simulink model "ADRC_ESO_feedback_comparison"  (R2020b)
settings: Solver=VariableStepAuto  StartTime=0.0  StopTime=10.0  RelTol=1e-3
values from neighbouring files (symbols this model uses):
  b = V*Km/(g*Tc^2*57.3)    [param_ADRC_ang_acc_change.m]
  b0 = -30    [param_ADRC_ang_acc_change.m]
  g = 9.81    [param_ADRC_ang_acc_change.m]
  g1 = 1/Tc^2    [param_ADRC_ang_acc_change.m]
  g2 = 2*Ac/Tc    [param_ADRC_ang_acc_change.m]
  kd = 2*wc*V/(g*57.3)    (= 21.3480207716)    [param_ADRC_ang_acc_change.m]
  kp = wc^2    (= 400)    [param_ADRC_ang_acc_change.m]
  V = 300    [param_ADRC_ang_acc_change.m]
  wo = 80    [param_ADRC_ang_acc_change.m]
settings Model: Creator=11814  LastModifiedBy=11814

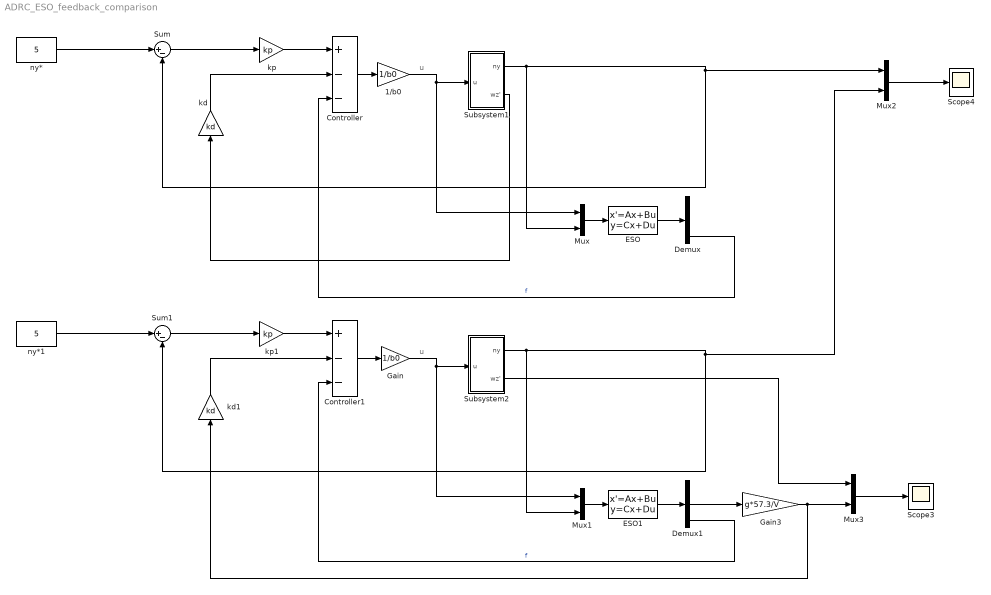
== system ADRC_ESO_feedback_comparison ==
  note: u
  note: u
  1/b0 : Gain  Gain=1/b0
  Controller : Sum  Inputs=+--
  Controller1 : Sum  Inputs=+--
  Demux : Demux  Outputs=3
  Demux1 : Demux  Outputs=3
  ESO : StateSpace  A=[-3*wo 1 0; -3*wo^2 0 1; -wo^3 0 0]  B=[0 3*wo; b0 3*wo^2; 0 wo^3]  C=eye(3)  D=[0 0; 0 0; 0 0]  InitialCondition=0
  ESO1 : StateSpace  A=[-3*wo 1 0; -3*wo^2 0 1; -wo^3 0 0]  B=[0 3*wo; b0 3*wo^2; 0 wo^3]  C=eye(3)  D=[0 0; 0 0; 0 0]  InitialCondition=0
  Gain : Gain  Gain=1/b0
  Gain3 : Gain  Gain=g*57.3/V
  Mux{,1..3} (4 alike) : Mux  Inputs=2
  Scope3 : Scope
  Scope4 : Scope
  Subsystem1 : Subsystem
  Subsystem2 : Subsystem
  Sum : Sum  Inputs=|+-
  Sum1 : Sum  Inputs=|+-
  kd : Gain  Gain=kd
  kd1 : Gain  Gain=kd
  kp : Gain  Gain=kp
  kp1 : Gain  Gain=kp
  ny* : Constant  Value=5
  ny*1 : Constant  Value=5
  wires:
  Controller/1 -> 1/b0/1
  ESO/1 -> Demux/1
  Demux/3 -> Controller/3  "f"
  ny*/1 -> Sum/1
  Mux/1 -> ESO/1
  Subsystem1/1(ny) -> Mux/2, Mux2/1, Sum/2
  kd/1 -> Controller/2
  Subsystem1/2(wz') -> kd/1
  kp/1 -> Controller/1
  Sum/1 -> kp/1
  1/b0/1 -> Mux/1, Subsystem1/1(u)
  Controller1/1 -> Gain/1
  ESO1/1 -> Demux1/1
  Demux1/3 -> Controller1/3  "f"
  ny*1/1 -> Sum1/1
  Mux1/1 -> ESO1/1
  Subsystem2/1(ny) -> Mux1/2, Mux2/2, Sum1/2
  kd1/1 -> Controller1/2
  kp1/1 -> Controller1/1
  Sum1/1 -> kp1/1
  Gain/1 -> Mux1/1, Subsystem2/1(u)
  Mux2/1 -> Scope4/1
  Mux3/1 -> Scope3/1
  Demux1/2 -> Gain3/1
  Gain3/1 -> Mux3/2, kd1/1
  Subsystem2/2(wz') -> Mux3/1

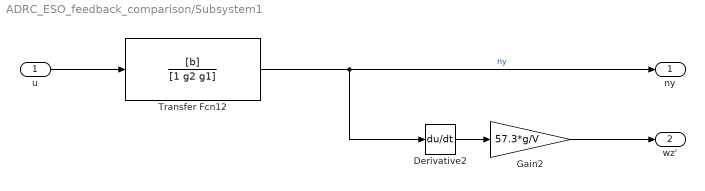
== system ADRC_ESO_feedback_comparison/Subsystem1 ==
  u : Inport
  Derivative2 : Derivative
  Gain2 : Gain  Gain=57.3*g/V
  Transfer Fcn12 : TransferFcn  Numerator=[b]  Denominator=[1 g2 g1]
  ny : Outport
  wz' : Outport  Port=2
  wires:
  u/1 -> Transfer Fcn12/1
  Transfer Fcn12/1 -> Derivative2/1, ny/1  "ny"
  Derivative2/1 -> Gain2/1
  Gain2/1 -> wz'/1

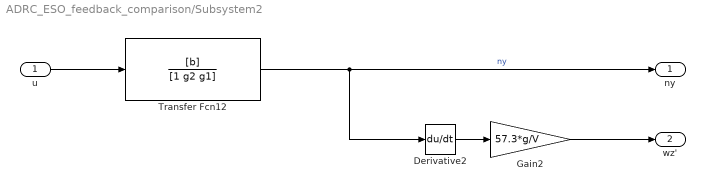
== system ADRC_ESO_feedback_comparison/Subsystem2 ==
  u : Inport
  Derivative2 : Derivative
  Gain2 : Gain  Gain=57.3*g/V
  Transfer Fcn12 : TransferFcn  Numerator=[b]  Denominator=[1 g2 g1]
  ny : Outport
  wz' : Outport  Port=2
  wires:
  u/1 -> Transfer Fcn12/1
  Transfer Fcn12/1 -> Derivative2/1, ny/1  "ny"
  Derivative2/1 -> Gain2/1
  Gain2/1 -> wz'/1
